simulink model "PiL_MARLUP_IAC26"  (R2026a)
settings: Solver=FixedStepDiscrete  StopTime=45  FixedStep=Ts  MaxStep=0.0025  RelTol=1e-4  AbsTol=1e-6  EnableMultiTasking=on
values from neighbouring files (symbols this model uses):
  A_obs = Ad*(eye(6) - L*Cd)    [Marlup_Final_Script.m]
  B_obs = [Bd, Ad*L]    [Marlup_Final_Script.m]
  C_obs = eye(6) - L*Cd    [Marlup_Final_Script.m]
  F_MAX = 1000    [Marlup_Final_Script.m]
  F_MIN = -1000    [Marlup_Final_Script.m]
  F_RATE = 1e5    (= 100000)    [Marlup_Final_Script.m]
  F_trim = [285.75; 271.60; 256.10]    [Marlup_Final_Script.m]
  K = dlqr(Ad, Bd, diag([2e4 2e3 2e4 2e3 4e3 4e2]), 1e-3*eye(3))    [Marlup_Final_Script.m]
  K_I = W \ (ki*eye(3))    [Marlup_Final_Script.m]
  L = Pp*Cd' / (Cd*Pp*Cd' + Rn)    [Marlup_Final_Script.m]    (also in graficar_marlup.m = textos(op.idioma); mediciones_marlup.m = L - mod(L,2))
  Ts = 0.01    [Marlup_Final_Script.m]
  x_obs0 = x_ref    [Marlup_Final_Script.m]
  y_ref = [0; 0; z0]    [Marlup_Final_Script.m]
  z0 = 1.571637930257020    (= 1.57163793026)    [Marlup_Final_Script.m]
undefined symbols (not defined in the file or in its folder): DiscIntNeverNeededParam
settings Model: Creator=Guerrero  LastModifiedBy=alvar
settings OptimizationCC: MaxStackSize=512
settings DebuggingCC: SubsystemReferenceDiagnosticForUnitTest=warning
settings HardwareCC: ProdLargestAtomicInteger=Long  ProdLargestAtomicFloat=Double  ProdHWDeviceType=ARM Compatible->ARM Cortex-M
settings RTWCC: SystemTargetFile=ert.tlc  HardwareBoard=STM32F4xx Based  TLCOptions=-aInlineSetEventsForThisBaseRateFcn=TLC_FALSE -aSuppressMultiTaskScheduler=TLC_FALSE -aRateBasedStepFcn=1  Toolchain=GNU Tools for STM32  BuildConfiguration=Faster Runs  Description=Embedded Coder
settings ERTTargetCC: ExtModeTransport=3.0  ExtModeStaticAllocSize=2048.0  CodeReplacementLibrary=ARM Cortex-M
settings SimscapeCC: SimscapeNominalValues="[{\"value\":\"1\",\"unit\":\"A\"},{\"value\":\"1\",\"unit\":\"bar\"},{\"value\":\"1\",\"unit\":\"cm^2\"},{\"value\":\"1\",\"unit\":\"cm^3/s\"},{\"value\":\"1\",\"unit\":\"kJ/kg\"},{\"value\":\"1\",\"unit\":\"kW\"},{\"value\":\"1\",\"unit\":\"l\"},{\"value\":\"1\",\"unit\":\"N\"},{\"value\":\"1\",\"unit\":\"N*m\"},{\"value\":\"1\",\"unit\":\"V\"}]"  SimscapeLogSimulationStatistics=on
settings ExplorerConfigSet: InternalSimMechanicsExplorerSettings=|
  | <ExplorerConfiguration>
  | 
  |   <canonicalview>default</canonicalview>
  | 
  |   <TilePanel>
  |     <TileInfo>
  |       <Tiles Columns="1" Count="1" Height="610" Rows="1" Width="1536">
  |         <Row Weight="1"/>
  |         <Column Weight="1"/>
  |         <Tile Height="1" Width="1" X="0" Y="0"/>
  |       </Tiles>
  |     </TileInfo>
  |     <SceneInfo>
  |       <SceneViewer>
  |         <IsThisViewStd>
  |           <IsStandardView>off</IsStandardView>
  |           <StandardViewName>Front</StandardViewName>
  |         </IsThisViewStd>
  |         <BGColor>
  |           <R>0.60000002384185791</R>
  |           <G>0.60000002384185791</G>
  |           <B>0.60000002384185791</B>
  |           <A>1</A>
  |         </BGColor>
  |         <Camera>
  |           <DoPerspective>off</DoPerspective>
  |           <Position>
  |             <X>1.7382</X>
  |             <Y>0.072429999999999994</Y>
  |             <Z>0.72370000000000001</Z>
  |           </Position>
  |           <Center>
  |             <X>-0.00779</X>
  |             <Y>0.072429999999999994</Y>
  |             <Z>0.72370000000000001</Z>
  |           </Center>
  |           <Up>
  |             <X>0</X>
  |             <Y>0</Y>
  |             <Z>1</Z>
  |           </Up>
  |           <XLim>3.2136172047138216</XLim>
  |           <YLim>0.87723854541778568</YLim>
  |           <ViewLimDist>0.01</ViewLimDist>
  |         </Camera>
  |       </SceneViewer>
  |     </SceneInfo>
  |   </TilePanel>
  | 
  |   <MechEditorPanel>
  |     <GfxPanelCameraMap/>
  |     <Cameras/>
  |     <VideoCreator>
  |       <IncludeTiles>All</IncludeTiles>
  |       <IncludeTime>on</IncludeTime>
  |       <IncludeWorldFrame>off</IncludeWorldFrame>
  |       <PlaybackSpeedRatio>1</PlaybackSpeedRatio>
  |       <FrameRate>30</FrameRate>
  |       <FrameSize>auto</FrameSize>
  |       <VideoFormat>MotionJPEGAVI</VideoFormat>
  |     </VideoCreator>
  |   </MechEditorPanel>
  | 
  |   <PlaybackSettings>
  |     <PlaybackSpeedFactor>4</PlaybackSpeedFactor>
  |   </PlaybackSettings>
  | 
  | </ExplorerConfiguration>

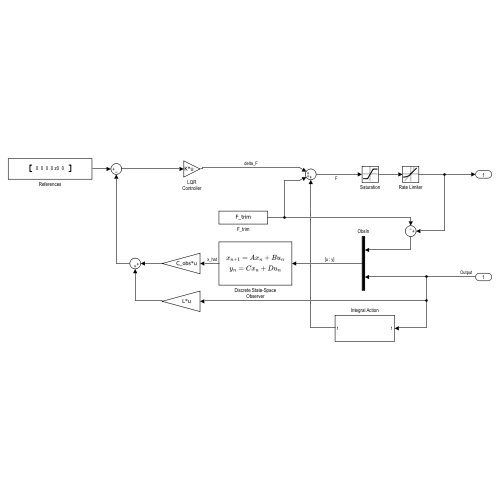
[thumbnail: Simulink's stored preview of the top-level diagram]
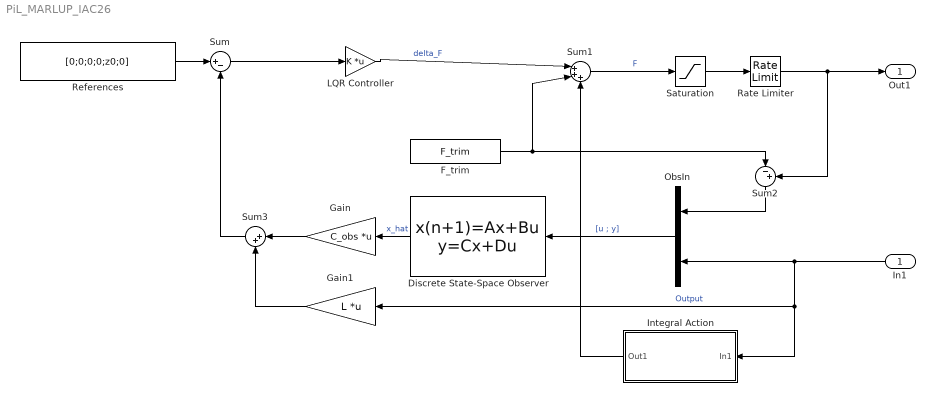
== system PiL_MARLUP_IAC26 ==
  In1 : Inport  OutDataTypeStr=double  PortDimensions=3  SampleTime=Ts
  Discrete State-Space Observer : DiscreteStateSpace  A=A_obs  B=B_obs  C=eye(6)  D=zeros(6,6)  InitialCondition=x_obs0  SampleTime=Ts
  F_trim : Constant  Value=F_trim
  Gain : Gain  Gain=C_obs  Multiplication=Matrix(K*u)
  Gain1 : Gain  Gain=L  Multiplication=Matrix(K*u)
  Integral Action : Subsystem
  LQR Controller : Gain  Gain=K  Multiplication=Matrix(K*u)
  ObsIn : Mux  Inputs=2
  Rate Limiter : RateLimiter  RisingSlewLimit=F_RATE  FallingSlewLimit=-F_RATE  SampleTimeMode=inherited
  References : Constant  Value=[0;0;0;0;z0;0]
  Saturation : Saturate  UpperLimit=F_MAX  LowerLimit=F_MIN  ZeroCross=off
  Sum : Sum  Inputs=|+-
  Sum1 : Sum  Inputs=|+++
  Sum2 : Sum  Inputs=|-+
  Sum3 : Sum  Inputs=|++
  Out1 : Outport  OutDataTypeStr=double  PortDimensions=3  SampleTime=Ts
  wires:
  Saturation/1 -> Rate Limiter/1
  In1/1 -> ObsIn/2, Integral Action/1(In1), Gain1/1  "Output"
  References/1 -> Sum/1
  LQR Controller/1 -> Sum1/1  "delta_F"
  Sum2/1 -> ObsIn/1
  ObsIn/1 -> Discrete State-Space Observer/1  "[u ; y]"
  F_trim/1 -> Sum2/1, Sum1/2
  Sum/1 -> LQR Controller/1
  Sum1/1 -> Saturation/1  "F"
  Discrete State-Space Observer/1 -> Gain/1  "x_hat"
  Rate Limiter/1 -> Out1/1, Sum2/2
  Integral Action/1(Out1) -> Sum1/3
  Gain/1 -> Sum3/1
  Gain1/1 -> Sum3/2
  Sum3/1 -> Sum/2

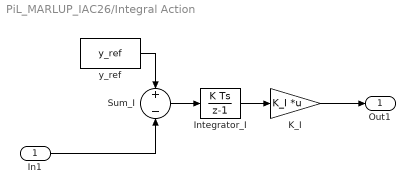
== system PiL_MARLUP_IAC26/Integral Action ==
  In1 : Inport  SampleTime=Ts
  Integrator_I : DiscreteIntegrator  SampleTime=Ts  ICPrevOutput=DiscIntNeverNeededParam  ICPrevScaledInput=DiscIntNeverNeededParam
  K_I : Gain  Gain=K_I  Multiplication=Matrix(K*u)
  Sum_I : Sum  Inputs=+-
  y_ref : Constant  Value=y_ref  SampleTime=Ts
  Out1 : Outport  SampleTime=Ts
  wires:
  In1/1 -> Sum_I/2
  Integrator_I/1 -> K_I/1
  y_ref/1 -> Sum_I/1
  Sum_I/1 -> Integrator_I/1
  K_I/1 -> Out1/1
